simulink model "deneme"  (R2019a)
settings: Solver=VariableStepAuto  StartTime=0.0  StopTime=10.0  RelTol=1e-3
settings Model: Creator=bilal  LastModifiedBy=bilal

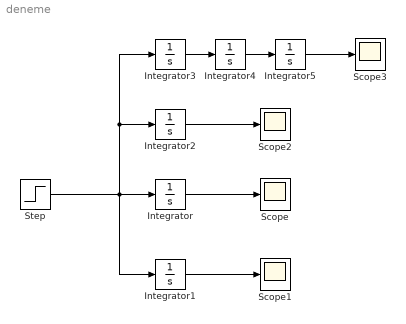
== system deneme ==
  Integrator{,1..5} (6 alike) : Integrator
  Scope{,1..3} (4 alike) : Scope
  Step : Step  SampleTime=0
  wires:
  Integrator/1 -> Scope/1
  Integrator1/1 -> Scope1/1
  Integrator2/1 -> Scope2/1
  Integrator3/1 -> Integrator4/1
  Step/1 -> Integrator2/1, Integrator3/1, Integrator1/1, Integrator/1
  Integrator4/1 -> Integrator5/1
  Integrator5/1 -> Scope3/1
